simulink model "gm_proj_model"  (R2025b)
settings: Solver=VariableStepDiscrete  StartTime=0.0  StopTime=10  FixedStep=0.2  RelTol=1e-3
libraries: hdlsllib x1
settings Model: Creator=vladc  LastModifiedBy=vladc
settings OptimizationCC: BlockReduction=off  ConditionallyExecuteInputs=off
settings DebuggingCC: InheritedTsInSrcMsg=none  SingleTaskRateTransMsg=error

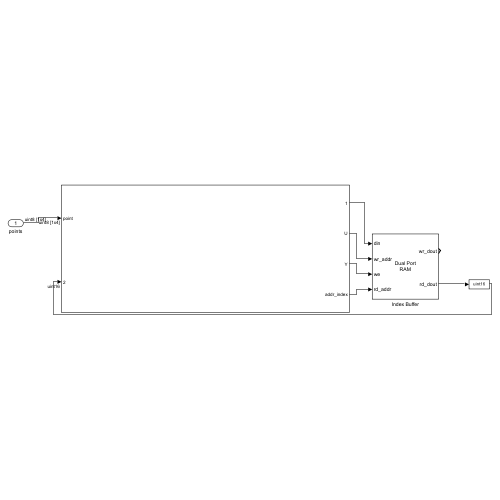
[thumbnail: Simulink's stored preview of the top-level diagram]
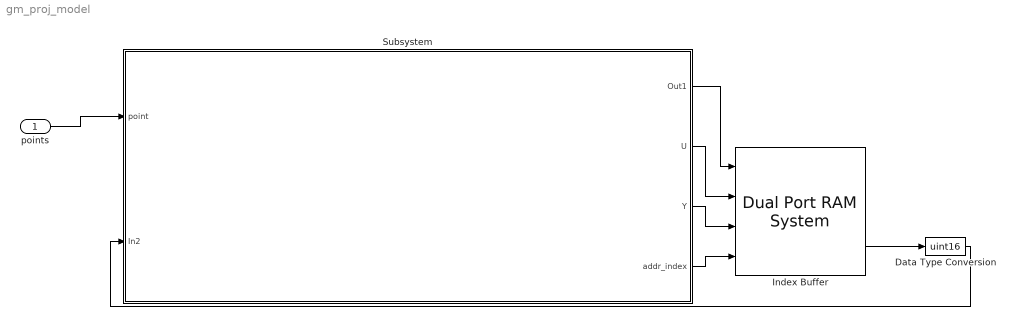
== system gm_proj_model ==
  points : Inport  OutDataTypeStr=uint8  PortDimensions=[1, 4]
  Data Type Conversion : DataTypeConversion  OutDataTypeStr=uint16  SaturateOnIntegerOverflow=off  RndMeth=Floor
  Index Buffer : hdlsllib/HDL RAMs/Dual Port RAM System  RAMType=Dual port  AsyncRead=off  WriteOutputValue=New data  RAMInitialValue=0  allowBusInputs=off  WritesHaveOutput=on  NumReads=0  NumWrites=1  SimulateUsing=Code generation  ModelRAMDelay=on  VectorAccess=Parallel
  Subsystem : Subsystem
  wires:
  Subsystem/4(addr_index) -> Index Buffer/4
  Subsystem/3(Y) -> Index Buffer/3
  Subsystem/2(U) -> Index Buffer/2
  Subsystem/1(Out1) -> Index Buffer/1
  Data Type Conversion/1 -> Subsystem/2(In2)
  points/1 -> Subsystem/1(point)
  Index Buffer/2 -> Data Type Conversion/1

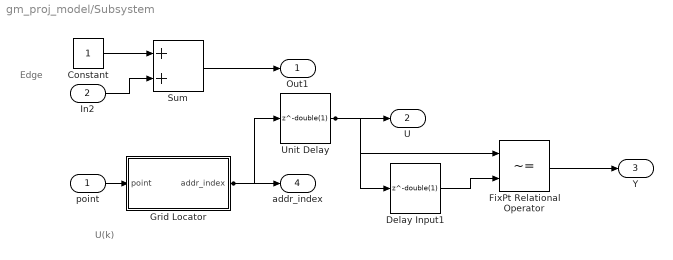
== system gm_proj_model/Subsystem ==
  note: Edge
  note: U(k)
  point : Inport  OutDataTypeStr=uint8  PortDimensions=[1 4]  SampleTime=0
  In2 : Inport  Port=2  OutDataTypeStr=uint16  PortDimensions=1  SampleTime=0
  Constant : Constant  OutDataTypeStr=uint16
  Delay Input1 : Delay  DelayLength=double(1)  InitialCondition=0  SampleTime=0.2
  FixPt Relational Operator : RelationalOperator  Operator=~=  OutDataTypeStr=boolean  SampleTime=0.2  InputSameDT=off
  Grid Locator : Subsystem
  Sum : Sum  OutDataTypeStr=uint16  AccumDataTypeStr=uint16
  Unit Delay : Delay  DelayLength=double(1)  InitialCondition=0  SampleTime=0.2
  Out1 : Outport
  U : Outport  Port=2  SampleTime=0.2
  Y : Outport  Port=3  SampleTime=0.2
  addr_index : Outport  Port=4  SampleTime=0
  wires:
  point/1 -> Grid Locator/1(point)
  In2/1 -> Sum/2
  Constant/1 -> Sum/1
  Unit Delay/1 -> FixPt Relational Operator/1, U/1, Delay Input1/1
  Sum/1 -> Out1/1
  Delay Input1/1 -> FixPt Relational Operator/2
  Grid Locator/1(addr_index) -> Unit Delay/1, addr_index/1
  FixPt Relational Operator/1 -> Y/1

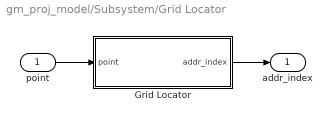
== system gm_proj_model/Subsystem/Grid Locator ==
  point : Inport  OutDataTypeStr=uint8  PortDimensions=[1 4]  SampleTime=0
  Grid Locator : MATLAB Function  TreatAsAtomicUnit=on
  addr_index : Outport  SampleTime=0  VectorParamsAs1DForOutWhenUnconnected=off
  wires:
  point/1 -> Grid Locator/1(point)
  Grid Locator/1(addr_index) -> addr_index/1

== matlab function gm_proj_model/Subsystem/Grid Locator/Grid Locator ==
  data: point input; addr_index output
function addr_index = getXY(point)
%#codegen
arguments
    point (1, 4) uint8
end

x = uint16(point(1));
y = uint16(point(2));

addr_index = (y * 256 + x) * 64 * 9;
